simulink model "distiller_controller"  (R2021a)
settings: Solver=VariableStepAuto  StartTime=0.0  StopTime=10.0  RelTol=1e-3
libraries: arduinolib x16
settings Model: Creator=Intuito_PC  LastModifiedBy=Intuito_PC

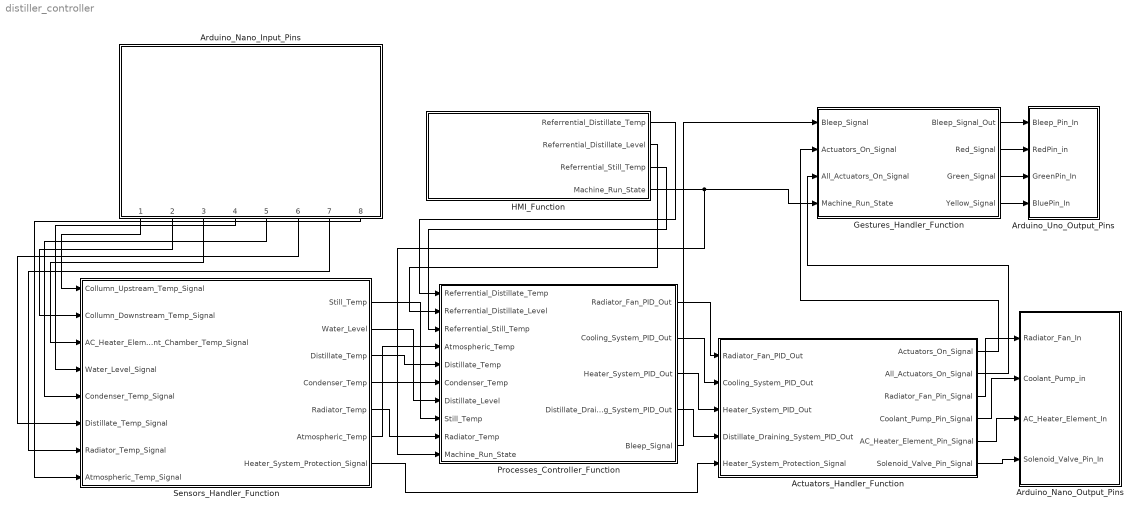
== system distiller_controller ==
  Actuators_Handler_Function : Subsystem
  Arduino_Nano_Input_Pins : Subsystem
  Arduino_Nano_Output_Pins : Subsystem
  Arduino_Uno_Output_Pins : Subsystem
  Gestures_Handler_Function : Subsystem
  HMI_Function : Subsystem
  Processes_Controller_Function : Subsystem
  Sensors_Handler_Function : Subsystem
  wires:
  Processes_Controller_Function/1(Radiator_Fan_PID_Out) -> Actuators_Handler_Function/1(Radiator_Fan_PID_Out)
  Processes_Controller_Function/2(Cooling_System_PID_Out) -> Actuators_Handler_Function/2(Cooling_System_PID_Out)
  Processes_Controller_Function/3(Heater_System_PID_Out) -> Actuators_Handler_Function/3(Heater_System_PID_Out)
  Processes_Controller_Function/4(Distillate_Draining_System_PID_Out) -> Actuators_Handler_Function/4(Distillate_Draining_System_PID_Out)
  Processes_Controller_Function/5(Bleep_Signal) -> Gestures_Handler_Function/1(Bleep_Signal)
  Actuators_Handler_Function/1(Actuators_On_Signal) -> Gestures_Handler_Function/2(Actuators_On_Signal)
  Actuators_Handler_Function/2(All_Actuators_On_Signal) -> Gestures_Handler_Function/3(All_Actuators_On_Signal)
  Sensors_Handler_Function/6(Atmospheric_Temp) -> Processes_Controller_Function/4(Atmospheric_Temp)
  Sensors_Handler_Function/7(Heater_System_Protection_Signal) -> Actuators_Handler_Function/5(Heater_System_Protection_Signal)
  Sensors_Handler_Function/5(Radiator_Temp) -> Processes_Controller_Function/9(Radiator_Temp)
  Sensors_Handler_Function/4(Condenser_Temp) -> Processes_Controller_Function/6(Condenser_Temp)
  Sensors_Handler_Function/3(Distillate_Temp) -> Processes_Controller_Function/5(Distillate_Temp)
  Sensors_Handler_Function/2(Water_Level) -> Processes_Controller_Function/7(Distillate_Level)
  Sensors_Handler_Function/1(Still_Temp) -> Processes_Controller_Function/8(Still_Temp)
  Gestures_Handler_Function/1(Bleep_Signal_Out) -> Arduino_Uno_Output_Pins/1(Bleep_Pin_In)
  Gestures_Handler_Function/2(Red_Signal) -> Arduino_Uno_Output_Pins/2(RedPin_in)
  Gestures_Handler_Function/3(Green_Signal) -> Arduino_Uno_Output_Pins/3(GreenPin_In)
  Gestures_Handler_Function/4(Yellow_Signal) -> Arduino_Uno_Output_Pins/4(BluePin_In)
  Actuators_Handler_Function/3(Radiator_Fan_Pin_Signal) -> Arduino_Nano_Output_Pins/1(Radiator_Fan_In)
  Actuators_Handler_Function/4(Coolant_Pump_Pin_Signal) -> Arduino_Nano_Output_Pins/2(Coolant_Pump_in)
  Actuators_Handler_Function/5(AC_Heater_Element_Pin_Signal) -> Arduino_Nano_Output_Pins/3(AC_Heater_Element_In)
  Actuators_Handler_Function/6(Solenoid_Valve_Pin_Signal) -> Arduino_Nano_Output_Pins/4(Solenoid_Valve_Pin_In)
  Arduino_Nano_Input_Pins/1(Collumn_Upstream_Temp_Signal) -> Sensors_Handler_Function/1(Collumn_Upstream_Temp_Signal)
  Arduino_Nano_Input_Pins/2(Collumn_Downstream_Temp_Signal) -> Sensors_Handler_Function/2(Collumn_Downstream_Temp_Signal)
  Arduino_Nano_Input_Pins/3(AC_Heater_Element_Chamber_Temp_Signal) -> Sensors_Handler_Function/3(AC_Heater_Element_Chamber_Temp_Signal)
  Arduino_Nano_Input_Pins/4(Water_Level_Signal) -> Sensors_Handler_Function/4(Water_Level_Signal)
  Arduino_Nano_Input_Pins/5(Condenser_Temp_Signal) -> Sensors_Handler_Function/5(Condenser_Temp_Signal)
  Arduino_Nano_Input_Pins/6(Distillate_Temp_Signal) -> Sensors_Handler_Function/6(Distillate_Temp_Signal)
  Arduino_Nano_Input_Pins/7(Radiator_Temp_Signal) -> Sensors_Handler_Function/7(Radiator_Temp_Signal)
  Arduino_Nano_Input_Pins/8(Atmospheric_Temp_Signal) -> Sensors_Handler_Function/8(Atmospheric_Temp_Signal)
  HMI_Function/4(Machine_Run_State) -> Processes_Controller_Function/10(Machine_Run_State), Gestures_Handler_Function/4(Machine_Run_State)
  HMI_Function/3(Referrential_Still_Temp) -> Processes_Controller_Function/3(Referrential_Still_Temp)
  HMI_Function/2(Referrential_Distillate_Level) -> Processes_Controller_Function/2(Referrential_Distillate_Level)
  HMI_Function/1(Referrential_Distillate_Temp) -> Processes_Controller_Function/1(Referrential_Distillate_Temp)

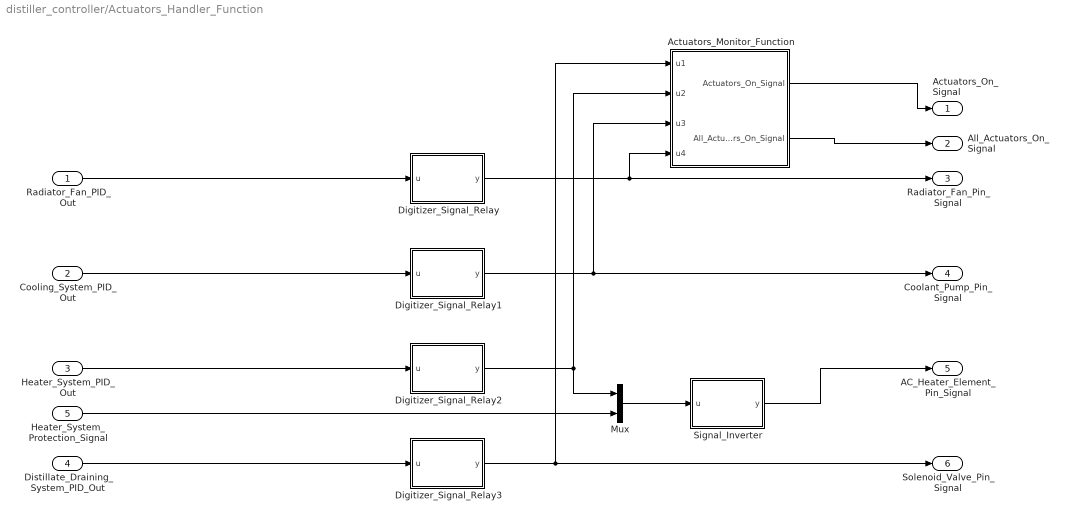
== system distiller_controller/Actuators_Handler_Function ==
  Radiator_Fan_PID_Out : Inport
  Cooling_System_PID_Out : Inport  Port=2
  Heater_System_PID_Out : Inport  Port=3
  Distillate_Draining_System_PID_Out : Inport  Port=4
  Heater_System_Protection_Signal : Inport  Port=5
  Actuators_Monitor_Function : MATLAB Function  TreatAsAtomicUnit=on
  Digitizer_Signal_Relay : MATLAB Function  TreatAsAtomicUnit=on
  Digitizer_Signal_Relay1 : MATLAB Function  TreatAsAtomicUnit=on
  Digitizer_Signal_Relay2 : MATLAB Function  TreatAsAtomicUnit=on
  Digitizer_Signal_Relay3 : MATLAB Function  TreatAsAtomicUnit=on
  Mux : Mux  Inputs=2
  Signal_Inverter : MATLAB Function  TreatAsAtomicUnit=on
  Actuators_On_Signal : Outport
  All_Actuators_On_Signal : Outport  Port=2
  Radiator_Fan_Pin_Signal : Outport  Port=3
  Coolant_Pump_Pin_Signal : Outport  Port=4
  AC_Heater_Element_Pin_Signal : Outport  Port=5
  Solenoid_Valve_Pin_Signal : Outport  Port=6
  wires:
  Digitizer_Signal_Relay2/1(y) -> Mux/1, Actuators_Monitor_Function/2(u2)
  Radiator_Fan_PID_Out/1 -> Digitizer_Signal_Relay/1(u)
  Cooling_System_PID_Out/1 -> Digitizer_Signal_Relay1/1(u)
  Heater_System_PID_Out/1 -> Digitizer_Signal_Relay2/1(u)
  Distillate_Draining_System_PID_Out/1 -> Digitizer_Signal_Relay3/1(u)
  Digitizer_Signal_Relay/1(y) -> Actuators_Monitor_Function/4(u4), Radiator_Fan_Pin_Signal/1
  Digitizer_Signal_Relay1/1(y) -> Actuators_Monitor_Function/3(u3), Coolant_Pump_Pin_Signal/1
  Signal_Inverter/1(y) -> AC_Heater_Element_Pin_Signal/1
  Digitizer_Signal_Relay3/1(y) -> Actuators_Monitor_Function/1(u1), Solenoid_Valve_Pin_Signal/1
  Actuators_Monitor_Function/1(Actuators_On_Signal) -> Actuators_On_Signal/1
  Actuators_Monitor_Function/2(All_Actuators_On_Signal) -> All_Actuators_On_Signal/1
  Mux/1 -> Signal_Inverter/1(u)
  Heater_System_Protection_Signal/1 -> Mux/2

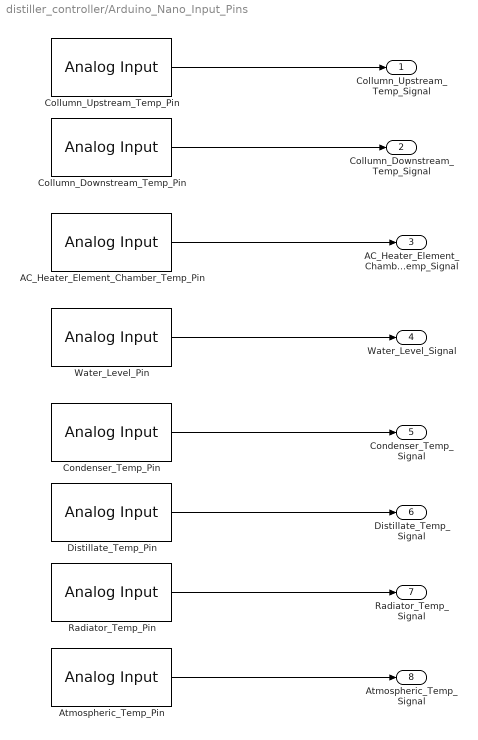
== system distiller_controller/Arduino_Nano_Input_Pins ==
  AC_Heater_Element_Chamber_Temp_Pin : arduinolib/Analog Input  pinNumber=4  ReadResultsOnly=off  ConversionTriggerSource=Software  ExternalTriggerType=uint32( 0 )  OutputDataType=uint16  EnableConversionCompleteNotify=off  EnableOuputStatus=off  SampleTime=-1  blockPlatform=arduino
  Atmospheric_Temp_Pin : arduinolib/Analog Input  pinNumber=4  ReadResultsOnly=off  ConversionTriggerSource=Software  ExternalTriggerType=uint32( 0 )  OutputDataType=uint16  EnableConversionCompleteNotify=off  EnableOuputStatus=off  SampleTime=-1  blockPlatform=arduino
  Collumn_Downstream_Temp_Pin : arduinolib/Analog Input  pinNumber=4  ReadResultsOnly=off  ConversionTriggerSource=Software  ExternalTriggerType=uint32( 0 )  OutputDataType=uint16  EnableConversionCompleteNotify=off  EnableOuputStatus=off  SampleTime=-1  blockPlatform=arduino
  Collumn_Upstream_Temp_Pin : arduinolib/Analog Input  pinNumber=4  ReadResultsOnly=off  ConversionTriggerSource=Software  ExternalTriggerType=uint32( 0 )  OutputDataType=uint16  EnableConversionCompleteNotify=off  EnableOuputStatus=off  SampleTime=-1  blockPlatform=arduino
  Condenser_Temp_Pin : arduinolib/Analog Input  pinNumber=4  ReadResultsOnly=off  ConversionTriggerSource=Software  ExternalTriggerType=uint32( 0 )  OutputDataType=uint16  EnableConversionCompleteNotify=off  EnableOuputStatus=off  SampleTime=-1  blockPlatform=arduino
  Distillate_Temp_Pin : arduinolib/Analog Input  pinNumber=4  ReadResultsOnly=off  ConversionTriggerSource=Software  ExternalTriggerType=uint32( 0 )  OutputDataType=uint16  EnableConversionCompleteNotify=off  EnableOuputStatus=off  SampleTime=-1  blockPlatform=arduino
  Radiator_Temp_Pin : arduinolib/Analog Input  pinNumber=4  ReadResultsOnly=off  ConversionTriggerSource=Software  ExternalTriggerType=uint32( 0 )  OutputDataType=uint16  EnableConversionCompleteNotify=off  EnableOuputStatus=off  SampleTime=-1  blockPlatform=arduino
  Water_Level_Pin : arduinolib/Analog Input  pinNumber=4  ReadResultsOnly=off  ConversionTriggerSource=Software  ExternalTriggerType=uint32( 0 )  OutputDataType=uint16  EnableConversionCompleteNotify=off  EnableOuputStatus=off  SampleTime=-1  blockPlatform=arduino
  Collumn_Upstream_Temp_Signal : Outport
  Collumn_Downstream_Temp_Signal : Outport  Port=2
  AC_Heater_Element_Chamber_Temp_Signal : Outport  Port=3
  Water_Level_Signal : Outport  Port=4
  Condenser_Temp_Signal : Outport  Port=5
  Distillate_Temp_Signal : Outport  Port=6
  Radiator_Temp_Signal : Outport  Port=7
  Atmospheric_Temp_Signal : Outport  Port=8
  wires:
  Collumn_Upstream_Temp_Pin/1 -> Collumn_Upstream_Temp_Signal/1
  Collumn_Downstream_Temp_Pin/1 -> Collumn_Downstream_Temp_Signal/1
  AC_Heater_Element_Chamber_Temp_Pin/1 -> AC_Heater_Element_Chamber_Temp_Signal/1
  Water_Level_Pin/1 -> Water_Level_Signal/1
  Condenser_Temp_Pin/1 -> Condenser_Temp_Signal/1
  Distillate_Temp_Pin/1 -> Distillate_Temp_Signal/1
  Radiator_Temp_Pin/1 -> Radiator_Temp_Signal/1
  Atmospheric_Temp_Pin/1 -> Atmospheric_Temp_Signal/1

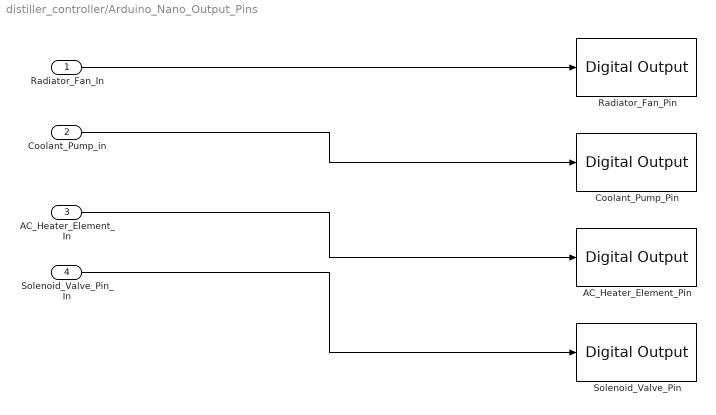
== system distiller_controller/Arduino_Nano_Output_Pins ==
  Radiator_Fan_In : Inport
  Coolant_Pump_in : Inport  Port=2
  AC_Heater_Element_In : Inport  Port=3
  Solenoid_Valve_Pin_In : Inport  Port=4
  AC_Heater_Element_Pin : arduinolib/Digital Output  pinNumber=5  Direction=output  blockPlatform=arduino
  Coolant_Pump_Pin : arduinolib/Digital Output  pinNumber=5  Direction=output  blockPlatform=arduino
  Radiator_Fan_Pin : arduinolib/Digital Output  pinNumber=5  Direction=output  blockPlatform=arduino
  Solenoid_Valve_Pin : arduinolib/Digital Output  pinNumber=5  Direction=output  blockPlatform=arduino
  wires:
  Coolant_Pump_in/1 -> Coolant_Pump_Pin/1
  Radiator_Fan_In/1 -> Radiator_Fan_Pin/1
  Solenoid_Valve_Pin_In/1 -> Solenoid_Valve_Pin/1
  AC_Heater_Element_In/1 -> AC_Heater_Element_Pin/1

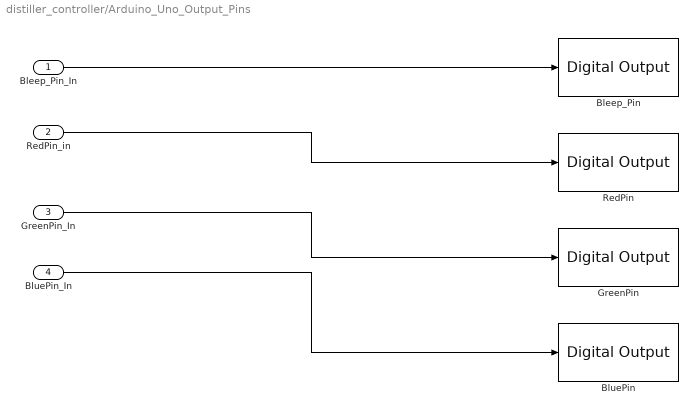
== system distiller_controller/Arduino_Uno_Output_Pins ==
  Bleep_Pin_In : Inport
  RedPin_in : Inport  Port=2
  GreenPin_In : Inport  Port=3
  BluePin_In : Inport  Port=4
  Bleep_Pin : arduinolib/Digital Output  pinNumber=5  Direction=output  blockPlatform=arduino
  BluePin : arduinolib/Digital Output  pinNumber=5  Direction=output  blockPlatform=arduino
  GreenPin : arduinolib/Digital Output  pinNumber=5  Direction=output  blockPlatform=arduino
  RedPin : arduinolib/Digital Output  pinNumber=5  Direction=output  blockPlatform=arduino
  wires:
  Bleep_Pin_In/1 -> Bleep_Pin/1
  RedPin_in/1 -> RedPin/1
  GreenPin_In/1 -> GreenPin/1
  BluePin_In/1 -> BluePin/1

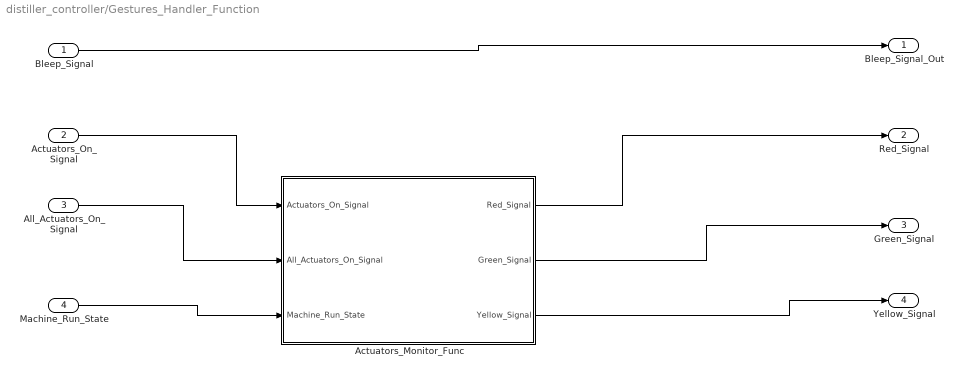
== system distiller_controller/Gestures_Handler_Function ==
  Bleep_Signal : Inport
  Actuators_On_Signal : Inport  Port=2
  All_Actuators_On_Signal : Inport  Port=3
  Machine_Run_State : Inport  Port=4
  Actuators_Monitor_Func : MATLAB Function  TreatAsAtomicUnit=on
  Bleep_Signal_Out : Outport
  Red_Signal : Outport  Port=2
  Green_Signal : Outport  Port=3
  Yellow_Signal : Outport  Port=4
  wires:
  Bleep_Signal/1 -> Bleep_Signal_Out/1
  Machine_Run_State/1 -> Actuators_Monitor_Func/3(Machine_Run_State)
  All_Actuators_On_Signal/1 -> Actuators_Monitor_Func/2(All_Actuators_On_Signal)
  Actuators_On_Signal/1 -> Actuators_Monitor_Func/1(Actuators_On_Signal)
  Actuators_Monitor_Func/1(Red_Signal) -> Red_Signal/1
  Actuators_Monitor_Func/2(Green_Signal) -> Green_Signal/1
  Actuators_Monitor_Func/3(Yellow_Signal) -> Yellow_Signal/1

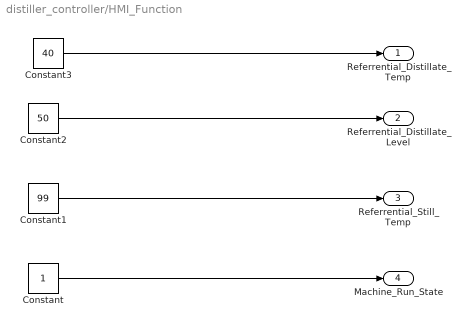
== system distiller_controller/HMI_Function ==
  Constant : Constant
  Constant1 : Constant  Value=99
  Constant2 : Constant  Value=50
  Constant3 : Constant  Value=40
  Referrential_Distillate_Temp : Outport
  Referrential_Distillate_Level : Outport  Port=2
  Referrential_Still_Temp : Outport  Port=3
  Machine_Run_State : Outport  Port=4
  wires:
  Constant/1 -> Machine_Run_State/1
  Constant3/1 -> Referrential_Distillate_Temp/1
  Constant2/1 -> Referrential_Distillate_Level/1
  Constant1/1 -> Referrential_Still_Temp/1

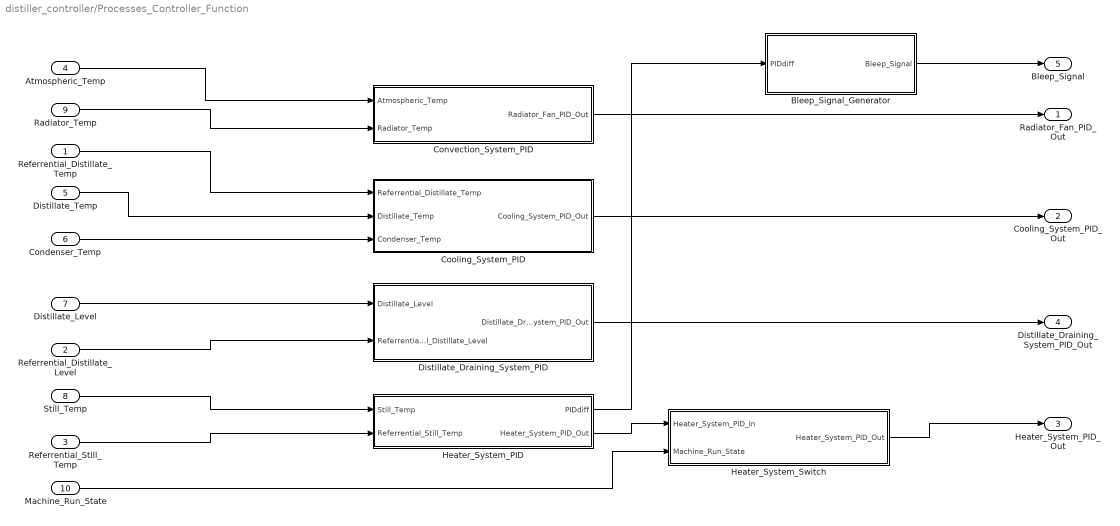
== system distiller_controller/Processes_Controller_Function ==
  Referrential_Distillate_Temp : Inport
  Referrential_Distillate_Level : Inport  Port=2
  Referrential_Still_Temp : Inport  Port=3
  Atmospheric_Temp : Inport  Port=4
  Distillate_Temp : Inport  Port=5
  Condenser_Temp : Inport  Port=6
  Distillate_Level : Inport  Port=7
  Still_Temp : Inport  Port=8
  Radiator_Temp : Inport  Port=9
  Machine_Run_State : Inport  Port=10
  Bleep_Signal_Generator : MATLAB Function  TreatAsAtomicUnit=on
  Convection_System_PID : MATLAB Function  TreatAsAtomicUnit=on
  Cooling_System_PID : MATLAB Function  TreatAsAtomicUnit=on
  Distillate_Draining_System_PID : MATLAB Function  TreatAsAtomicUnit=on
  Heater_System_PID : MATLAB Function  TreatAsAtomicUnit=on
  Heater_System_Switch : MATLAB Function  TreatAsAtomicUnit=on
  Radiator_Fan_PID_Out : Outport
  Cooling_System_PID_Out : Outport  Port=2
  Heater_System_PID_Out : Outport  Port=3
  Distillate_Draining_System_PID_Out : Outport  Port=4
  Bleep_Signal : Outport  Port=5
  wires:
  Heater_System_PID/2(Heater_System_PID_Out) -> Heater_System_Switch/1(Heater_System_PID_In)
  Heater_System_Switch/1(Heater_System_PID_Out) -> Heater_System_PID_Out/1
  Cooling_System_PID/1(Cooling_System_PID_Out) -> Cooling_System_PID_Out/1
  Convection_System_PID/1(Radiator_Fan_PID_Out) -> Radiator_Fan_PID_Out/1
  Distillate_Draining_System_PID/1(Distillate_Draining_System_PID_Out) -> Distillate_Draining_System_PID_Out/1
  Atmospheric_Temp/1 -> Convection_System_PID/1(Atmospheric_Temp)
  Radiator_Temp/1 -> Convection_System_PID/2(Radiator_Temp)
  Referrential_Distillate_Temp/1 -> Cooling_System_PID/1(Referrential_Distillate_Temp)
  Distillate_Temp/1 -> Cooling_System_PID/2(Distillate_Temp)
  Condenser_Temp/1 -> Cooling_System_PID/3(Condenser_Temp)
  Distillate_Level/1 -> Distillate_Draining_System_PID/1(Distillate_Level)
  Referrential_Distillate_Level/1 -> Distillate_Draining_System_PID/2(Referrential_Distillate_Level)
  Still_Temp/1 -> Heater_System_PID/1(Still_Temp)
  Referrential_Still_Temp/1 -> Heater_System_PID/2(Referrential_Still_Temp)
  Machine_Run_State/1 -> Heater_System_Switch/2(Machine_Run_State)
  Heater_System_PID/1(PIDdiff) -> Bleep_Signal_Generator/1(PIDdiff)
  Bleep_Signal_Generator/1(Bleep_Signal) -> Bleep_Signal/1

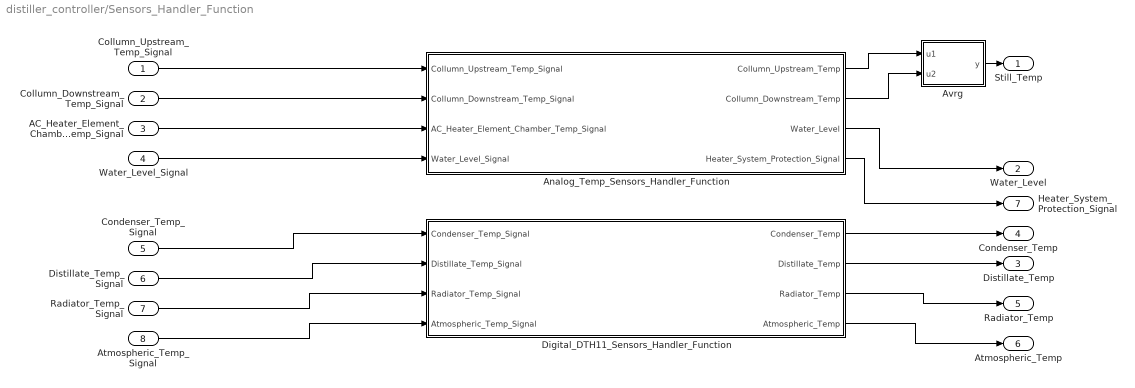
== system distiller_controller/Sensors_Handler_Function ==
  Collumn_Upstream_Temp_Signal : Inport
  Collumn_Downstream_Temp_Signal : Inport  Port=2
  AC_Heater_Element_Chamber_Temp_Signal : Inport  Port=3
  Water_Level_Signal : Inport  Port=4
  Condenser_Temp_Signal : Inport  Port=5
  Distillate_Temp_Signal : Inport  Port=6
  Radiator_Temp_Signal : Inport  Port=7
  Atmospheric_Temp_Signal : Inport  Port=8
  Analog_Temp_Sensors_Handler_Function : MATLAB Function  TreatAsAtomicUnit=on
  Avrg : MATLAB Function  TreatAsAtomicUnit=on
  Digital_DTH11_Sensors_Handler_Function : MATLAB Function  TreatAsAtomicUnit=on
  Still_Temp : Outport
  Water_Level : Outport  Port=2
  Distillate_Temp : Outport  Port=3
  Condenser_Temp : Outport  Port=4
  Radiator_Temp : Outport  Port=5
  Atmospheric_Temp : Outport  Port=6
  Heater_System_Protection_Signal : Outport  Port=7
  wires:
  Condenser_Temp_Signal/1 -> Digital_DTH11_Sensors_Handler_Function/1(Condenser_Temp_Signal)
  Distillate_Temp_Signal/1 -> Digital_DTH11_Sensors_Handler_Function/2(Distillate_Temp_Signal)
  Radiator_Temp_Signal/1 -> Digital_DTH11_Sensors_Handler_Function/3(Radiator_Temp_Signal)
  Atmospheric_Temp_Signal/1 -> Digital_DTH11_Sensors_Handler_Function/4(Atmospheric_Temp_Signal)
  Water_Level_Signal/1 -> Analog_Temp_Sensors_Handler_Function/4(Water_Level_Signal)
  AC_Heater_Element_Chamber_Temp_Signal/1 -> Analog_Temp_Sensors_Handler_Function/3(AC_Heater_Element_Chamber_Temp_Signal)
  Collumn_Downstream_Temp_Signal/1 -> Analog_Temp_Sensors_Handler_Function/2(Collumn_Downstream_Temp_Signal)
  Collumn_Upstream_Temp_Signal/1 -> Analog_Temp_Sensors_Handler_Function/1(Collumn_Upstream_Temp_Signal)
  Digital_DTH11_Sensors_Handler_Function/1(Condenser_Temp) -> Condenser_Temp/1
  Digital_DTH11_Sensors_Handler_Function/2(Distillate_Temp) -> Distillate_Temp/1
  Digital_DTH11_Sensors_Handler_Function/3(Radiator_Temp) -> Radiator_Temp/1
  Digital_DTH11_Sensors_Handler_Function/4(Atmospheric_Temp) -> Atmospheric_Temp/1
  Analog_Temp_Sensors_Handler_Function/3(Water_Level) -> Water_Level/1
  Analog_Temp_Sensors_Handler_Function/4(Heater_System_Protection_Signal) -> Heater_System_Protection_Signal/1
  Avrg/1(y) -> Still_Temp/1
  Analog_Temp_Sensors_Handler_Function/1(Collumn_Upstream_Temp) -> Avrg/1(u1)
  Analog_Temp_Sensors_Handler_Function/2(Collumn_Downstream_Temp) -> Avrg/2(u2)

== matlab function distiller_controller/Gestures_Handler_Function/Actuators_Monitor_Func ==
  data: Actuators_On_Signal input; Red_Signal output; All_Actuators_On_Signal input; Machine_Run_State input; Green_Signal output; Yellow_Signal output
function [Red_Signal, Green_Signal, Yellow_Signal] = fcn(Actuators_On_Signal, All_Actuators_On_Signal, Machine_Run_State)
if Actuators_On_Signal > 0
%     Light yellow
        Yellow_Signal = 1;
else
    %     Light yellow off
        Yellow_Signal = 0;
end
if All_Actuators_On_Signal > 0
%     Light Red
        Red_Signal = 1;
else
    %     Light Red off
        Red_Signal = 0;
end
if Machine_Run_State == 0
%     Light Green in standby
        Green_Signal = 1;
else
    %     Light yellow oof
        Green_Signal = 0;
end
end

== matlab function distiller_controller/Sensors_Handler_Function/Analog_Temp_Sensors_Handler_Function ==
  data: Collumn_Upstream_Temp_Signal input; Collumn_Upstream_Temp output; Collumn_Downstream_Temp_Signal input; AC_Heater_Element_Chamber_Temp_Signal input; Water_Level_Signal input; Collumn_Downstream_Temp output; Water_Level output; Heater_System_Protection_Signal output
function [Collumn_Upstream_Temp, Collumn_Downstream_Temp, Water_Level, Heater_System_Protection_Signal] = fcn(Collumn_Upstream_Temp_Signal, Collumn_Downstream_Temp_Signal, AC_Heater_Element_Chamber_Temp_Signal, Water_Level_Signal)
% Analog Temp Sensors Constants
THERMISTORNOMINAL = 90000;
TEMPERATURENOMINAL = 298; % 25 dge_C
BCOEFFICIENT = 3950;
SERIESRESISTOR = 10000; % R_1

% Temp sensor 1
R_1 = double(SERIESRESISTOR*(Collumn_Upstream_Temp_Signal/1023)/(5 - (Collumn_Upstream_Temp_Signal/1023)*4.99)); % NTC Resistance
Collumn_Upstream_Temp = 1/(1/TEMPERATURENOMINAL - log(abs(THERMISTORNOMINAL/R_1))/BCOEFFICIENT) -273; % Compute temp
% Temp sensor 2
R_2 = double(SERIESRESISTOR*(Collumn_Downstream_Temp_Signal/1023)/(5 - (Collumn_Downstream_Temp_Signal/1023)*4.99)); % NTC Resistance
Collumn_Downstream_Temp = 1/(1/TEMPERATURENOMINAL - log(abs(THERMISTORNOMINAL/R_2))/BCOEFFICIENT) -273; % Compute temp
% Temp sensor 3
R_3 = double(SERIESRESISTOR*(AC_Heater_Element_Chamber_Temp_Signal/1023)/(5 - (AC_Heater_Element_Chamber_Temp_Signal/1023)*4.99)); % NTC Resistance
AC_Heater_Element_Chamber_Temp = 1/(1/TEMPERATURENOMINAL - log(abs(THERMISTORNOMINAL/R_3))/BCOEFFICIENT) -273; % Compute temp

% Water level sensor
Water_Level = double(Water_Level_Signal/1023*100);

% Heater System Protection
if AC_Heater_Element_Chamber_Temp > 160
    Heater_System_Protection_Signal = 1;
else
    Heater_System_Protection_Signal = 0;
end
end

== matlab function distiller_controller/Sensors_Handler_Function/Digital_DTH11_Sensors_Handler_Function ==
  data: Condenser_Temp_Signal input; Condenser_Temp output; Distillate_Temp_Signal input; Radiator_Temp_Signal input; Atmospheric_Temp_Signal input; Distillate_Temp output; Radiator_Temp output; Atmospheric_Temp output
function [Condenser_Temp, Distillate_Temp, Radiator_Temp, Atmospheric_Temp] = fcn(Condenser_Temp_Signal, Distillate_Temp_Signal, Radiator_Temp_Signal, Atmospheric_Temp_Signal)
% Analog Temp Sensors Constants
THERMISTORNOMINAL = 90000;
TEMPERATURENOMINAL = 298; % 25 dge_C
BCOEFFICIENT = 3950;
SERIESRESISTOR = 10000; % R_1

% Temp sensor 1
R_1 = double(SERIESRESISTOR*(Condenser_Temp_Signal/1023)/(5 - (Condenser_Temp_Signal/1023)*4.99)); % NTC Resistance
Condenser_Temp = 1/(1/TEMPERATURENOMINAL - log(abs(THERMISTORNOMINAL/R_1))/BCOEFFICIENT) -273; % Compute temp
% Temp sensor 2
R_2 = double(SERIESRESISTOR*(Distillate_Temp_Signal/1023)/(5 - (Distillate_Temp_Signal/1023)*4.99)); % NTC Resistance
Distillate_Temp = 1/(1/TEMPERATURENOMINAL - log(abs(THERMISTORNOMINAL/R_2))/BCOEFFICIENT) -273; % Compute temp
% Temp sensor 3
R_3 = double(SERIESRESISTOR*(Radiator_Temp_Signal/1023)/(5 - (Radiator_Temp_Signal/1023)*4.99)); % NTC Resistance
Radiator_Temp = 1/(1/TEMPERATURENOMINAL - log(abs(THERMISTORNOMINAL/R_3))/BCOEFFICIENT) -273; % Compute temp
% Temp sensor 4
R_4 = double(SERIESRESISTOR*(Atmospheric_Temp_Signal/1023)/(5 - (Atmospheric_Temp_Signal/1023)*4.99)); % NTC Resistance
Atmospheric_Temp = 1/(1/TEMPERATURENOMINAL - log(abs(THERMISTORNOMINAL/R_4))/BCOEFFICIENT) -273; % Compute temp
end

== matlab function distiller_controller/Sensors_Handler_Function/Avrg ==
  data: u1 input; y output; u2 input
function y = fcn(u1, u2)
% Average
y = (u1 + u2)/2;
end

== matlab function distiller_controller/Processes_Controller_Function/Cooling_System_PID ==
  data: Referrential_Distillate_Temp input; Cooling_System_PID_Out output; Distillate_Temp input; Condenser_Temp input
function Cooling_System_PID_Out = fcn(Referrential_Distillate_Temp, Distillate_Temp, Condenser_Temp)
% PID Constants
kP = 0.1; %Proportinal Constant
kI = 2;  %Integral Constant
kD = 0.5;  %Differential Constant
% Compute PID Control
PIDdiff = ((Distillate_Temp + Condenser_Temp)/2 - Referrential_Distillate_Temp);
PIDintegral =+ PIDdiff ;
Cooling_System_PID_Out = kP*PIDdiff + kI*PIDintegral+ kD;
end

== matlab function distiller_controller/Processes_Controller_Function/Convection_System_PID ==
  data: Atmospheric_Temp input; Radiator_Fan_PID_Out output; Radiator_Temp input
function Radiator_Fan_PID_Out = fcn(Atmospheric_Temp, Radiator_Temp)
% PID Constants
kP = 0.1; %Proportinal Constant
kI = 2;  %Integral Constant
kD = 0.5;  %Differential Constant
% Compute PID Control
PIDdiff = (Radiator_Temp - Atmospheric_Temp);
PIDintegral =+ PIDdiff ;
Radiator_Fan_PID_Out = kP*PIDdiff + kI*PIDintegral + kD;
end

== matlab function distiller_controller/Processes_Controller_Function/Heater_System_PID ==
  data: PIDdiff output; Still_Temp input; Heater_System_PID_Out output; Referrential_Still_Temp input
function [PIDdiff, Heater_System_PID_Out] = fcn(Still_Temp, Referrential_Still_Temp)
% PID Constants
kP = 0.1; %Proportinal Constant
kI = 2;  %Integral Constant
kD = 0.5;  %Differential Constant
% Compute PID Control
PIDdiff = (Referrential_Still_Temp - Still_Temp);
PIDintegral =+ PIDdiff ;
Heater_System_PID_Out = kP*PIDdiff + kI*PIDintegral + kD;
end

== matlab function distiller_controller/Processes_Controller_Function/Distillate_Draining_System_PID ==
  data: Distillate_Level input; Distillate_Draining_System_PID_Out output; Referrential_Distillate_Level input
function Distillate_Draining_System_PID_Out = fcn(Distillate_Level, Referrential_Distillate_Level)
% PID Constants
kP = 0.1; %Proportinal Constant
kI = 2;  %Integral Constant
kD = 0.5;  %Differential Constant
% Compute PID Control
PIDdiff = (Referrential_Distillate_Level - Distillate_Level);
PIDintegral =+ PIDdiff ;
Distillate_Draining_System_PID_Out = kP*PIDdiff + kI*PIDintegral + kD;
end

== matlab function distiller_controller/Processes_Controller_Function/Heater_System_Switch ==
  data: Heater_System_PID_In input; Heater_System_PID_Out output; Machine_Run_State input
function Heater_System_PID_Out = fcn(Heater_System_PID_In, Machine_Run_State)
% Check Machine Run State
if Machine_Run_State == 1  % “Standby”, “Running” : (0, 1)
    Heater_System_PID_Out = Heater_System_PID_In; % ON Value
else 
    Heater_System_PID_Out = 0; % OFF Value
end

== matlab function distiller_controller/Actuators_Handler_Function/Digitizer_Signal_Relay ==
  data: u input; y output
function y = fcn(u)
% Define limit
limit = 30;
if u > limit
    y = 1;
else
    y = 0;
end
end

== matlab function distiller_controller/Actuators_Handler_Function/Signal_Inverter ==
  data: u input; y output
function y = fcn(u)
% Invert the input
if u == 1
    y = 0;
else
    y = 1;
end
end

== matlab function distiller_controller/Actuators_Handler_Function/Digitizer_Signal_Relay1 ==
  data: u input; y output
function y = fcn(u)
% Define limit
limit = 30;
if u > limit
    y = 1;
else
    y = 0;
end
end

== matlab function distiller_controller/Actuators_Handler_Function/Digitizer_Signal_Relay2 ==
  data: u input; y output
function y = fcn(u)
% Define limit
limit = 30;
if u > limit
    y = 1;
else
    y = 0;
end
end

== matlab function distiller_controller/Actuators_Handler_Function/Digitizer_Signal_Relay3 ==
  data: u input; y output
function y = fcn(u)
% Define limit
limit = 30;
if u > limit
    y = 1;
else
    y = 0;
end
end

== matlab function distiller_controller/Processes_Controller_Function/Bleep_Signal_Generator ==
  data: PIDdiff input; Bleep_Signal output
function Bleep_Signal = fcn(PIDdiff)
% Trigger the buzzer on accurate heating
if abs(PIDdiff) < 1
    pause(1); %pause for 1 sec
    Bleep_Signal = 1;
    pause(1); %pause for 1 sec
else
    Bleep_Signal = 0;
end
end

== matlab function distiller_controller/Actuators_Handler_Function/Actuators_Monitor_Function ==
  data: u1 input; Actuators_On_Signal output; u2 input; u3 input; u4 input; All_Actuators_On_Signal output
function [Actuators_On_Signal, All_Actuators_On_Signal] = fcn(u1, u2, u3, u4)
% Initiate defaults
Actuators_On_Signal = 0;
All_Actuators_On_Signal = 0;
% Check actuators switch states
if (u1 + u2 + u3 + u4) < 1 
%     All_Actuators_On_Signal = 0; % Check if all actuators are on
    Actuators_On_Signal = 0; 
elseif (u1 + u2 + u3 + u4) > 0 && (u1 + u2 + u3 + u4) <= 3.1 
    Actuators_On_Signal = 1; % Check if an actuator is on
end
    if (u1 + u2 + u3 + u4) > 3.5
    All_Actuators_On_Signal = 1; % Check if all actuators are on
    else
       All_Actuators_On_Signal = 0; % Check if all actuators are on
end
end
